simulink model "Cascade_form"  (R2020b)
settings: Solver=VariableStepAuto  StartTime=0.0  StopTime=10.0  RelTol=1e-3
settings Model: Creator=Shivashis  LastModifiedBy=Shivashis
settings DataIOCC: SaveOutput=off  SaveTime=off

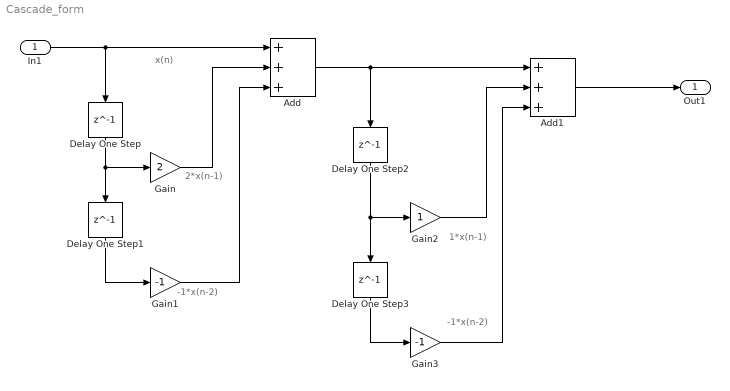
== system Cascade_form ==
  note: 1*x(n-1)
  note: -1*x(n-2)
  note: 2*x(n-1)
  note: x(n)
  note: -1*x(n-2)
  In1 : Inport  OutDataTypeStr=double  PortDimensions=1  SampleTime=0
  Add : Sum  Inputs=+++
  Add1 : Sum  Inputs=+++
  Delay One Step{,1..3} (4 alike) : Delay  DelayLength=1
  Gain : Gain  Gain=2
  Gain1 : Gain  Gain=-1
  Gain2 : Gain
  Gain3 : Gain  Gain=-1
  Out1 : Outport  OutDataTypeStr=double  PortDimensions=1  SampleTime=0
  wires:
  Gain3/1 -> Add1/3
  Delay One Step3/1 -> Gain3/1
  Delay One Step2/1 -> Gain2/1, Delay One Step3/1
  Delay One Step1/1 -> Gain1/1
  Add/1 -> Add1/1, Delay One Step2/1
  Delay One Step/1 -> Delay One Step1/1, Gain/1
  Gain2/1 -> Add1/2
  In1/1 -> Add/1, Delay One Step/1
  Gain/1 -> Add/2
  Gain1/1 -> Add/3
  Add1/1 -> Out1/1
